simulink model "Lookup_verif"  (Simulink 7.2)
settings: Solver=ode45  StartTime=0.0  StopTime=10.0  RelTol=1e-3
settings Model: Creator=Romain  LastModifiedBy=Romain
settings OptimizationCC: ExpressionDepthLimit=128
settings DebuggingCC: SolverPrmCheckMsg=none  FcnCallInpInsideContextMsg=Enable All  StateNameClashWarn=none  StrictBusMsg=ErrorLevel1
settings CodeAppCC: CustomSymbolStrType=$N$R$M_T
settings GRTTargetCC: TargetFunctionLibrary=C89/C90 (ANSI)

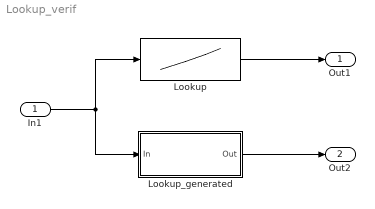
== system Lookup_verif ==
  In1 : Inport  OutDataTypeStr=double  DataType=double
  Lookup : Lookup  RequirementInfo={} %GIDa_7e2db0e9_94b6_4bd9_a9f6_4e499dfb9412  InputValues=[0 120 350 500]  Table=[1.0 1.0 0.3 0.3]
  Lookup_generated : Subsystem  TreatAsAtomicUnit=on
  Out1 : Outport
  Out2 : Outport  Port=2
  wires:
  In1/1 -> Lookup_generated/1(In), Lookup/1
  Lookup/1 -> Out1/1
  Lookup_generated/1(Out) -> Out2/1

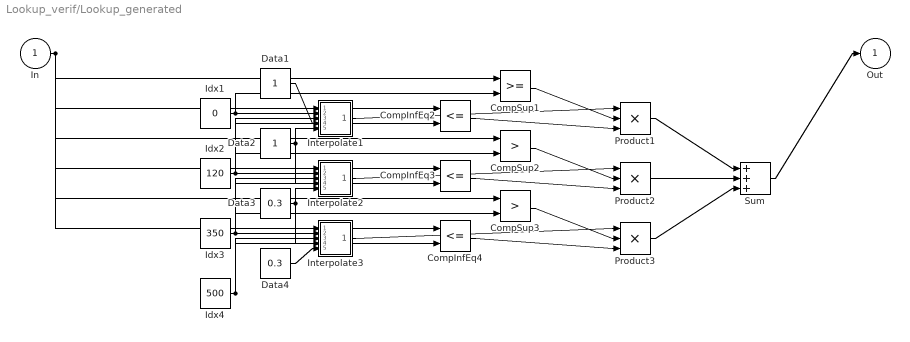
== system Lookup_verif/Lookup_generated ==
  In : Inport
  CompInfEq2 : RelationalOperator  Operator=<=  InputSameDT=on
  CompInfEq3 : RelationalOperator  Operator=<=  InputSameDT=on
  CompInfEq4 : RelationalOperator  Operator=<=  InputSameDT=on
  CompSup1 : RelationalOperator  InputSameDT=on
  CompSup2 : RelationalOperator  Operator=>  InputSameDT=on
  CompSup3 : RelationalOperator  Operator=>  InputSameDT=on
  Data1 : Constant
  Data2 : Constant
  Data3 : Constant  Value=0.3
  Data4 : Constant  Value=0.3
  Idx1 : Constant  Value=0
  Idx2 : Constant  Value=120
  Idx3 : Constant  Value=350
  Idx4 : Constant  Value=500
  Interpolate1 : Subsystem  TreatAsAtomicUnit=on
  Interpolate2 : Subsystem  TreatAsAtomicUnit=on
  Interpolate3 : Subsystem  TreatAsAtomicUnit=on
  Product1 : Product  Inputs=***  SaturateOnIntegerOverflow=on  RndMeth=Zero  OutDataTypeStr=Inherit: Same as first input
  Product2 : Product  Inputs=***  SaturateOnIntegerOverflow=on  RndMeth=Zero  OutDataTypeStr=Inherit: Same as first input
  Product3 : Product  Inputs=***  SaturateOnIntegerOverflow=on  RndMeth=Zero  OutDataTypeStr=Inherit: Same as first input
  Sum : Sum  Inputs=+++  SaturateOnIntegerOverflow=on  InputSameDT=on  OutDataTypeStr=Inherit: Same as first input
  Out : Outport
  wires:
  In/1 -> Interpolate1/1(InportIn), CompSup1/1, Interpolate2/1(InportIn), CompSup2/1, CompInfEq2/1, Interpolate3/1(InportIn), CompSup3/1, CompInfEq3/1, CompInfEq4/1
  Idx1/1 -> Interpolate1/2(InportIdx1), CompSup1/2
  Data1/1 -> Interpolate1/4(InportData1)
  Interpolate1/1(Out) -> Product1/1
  CompSup1/1 -> Product1/2
  CompInfEq2/1 -> Product1/3
  Product1/1 -> Sum/1
  Idx2/1 -> Interpolate2/2(InportIdx1), CompSup2/2, Interpolate1/3(InportIdx2), CompInfEq2/2
  Data2/1 -> Interpolate2/4(InportData1), Interpolate1/5(InportData2)
  Interpolate2/1(Out) -> Product2/1
  CompSup2/1 -> Product2/2
  CompInfEq3/1 -> Product2/3
  Product2/1 -> Sum/2
  Idx3/1 -> Interpolate3/2(InportIdx1), CompSup3/2, Interpolate2/3(InportIdx2), CompInfEq3/2
  Data3/1 -> Interpolate3/4(InportData1), Interpolate2/5(InportData2)
  Interpolate3/1(Out) -> Product3/1
  CompSup3/1 -> Product3/2
  CompInfEq4/1 -> Product3/3
  Product3/1 -> Sum/3
  Idx4/1 -> Interpolate3/3(InportIdx2), CompInfEq4/2
  Data4/1 -> Interpolate3/5(InportData2)
  Sum/1 -> Out/1

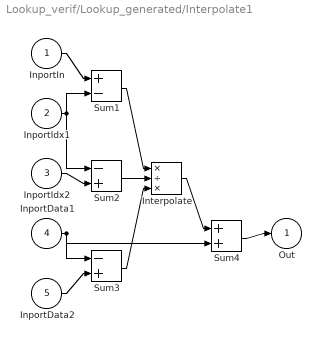
== system Lookup_verif/Lookup_generated/Interpolate1 ==
  InportIn : Inport
  InportIdx1 : Inport  Port=2
  InportIdx2 : Inport  Port=3
  InportData1 : Inport  Port=4
  InportData2 : Inport  Port=5
  Interpolate : Product  Inputs=*/*  SaturateOnIntegerOverflow=on  RndMeth=Zero  InputSameDT=on  OutDataTypeStr=Inherit: Same as first input
  Sum1 : Sum  Inputs=+-  SaturateOnIntegerOverflow=on  InputSameDT=on  OutDataTypeStr=Inherit: Same as first input
  Sum2 : Sum  Inputs=-+  SaturateOnIntegerOverflow=on  InputSameDT=on  OutDataTypeStr=Inherit: Same as first input
  Sum3 : Sum  Inputs=-+  SaturateOnIntegerOverflow=on  InputSameDT=on  OutDataTypeStr=Inherit: Same as first input
  Sum4 : Sum  SaturateOnIntegerOverflow=on  InputSameDT=on  OutDataTypeStr=Inherit: Same as first input
  Out : Outport
  wires:
  InportIn/1 -> Sum1/1
  InportIdx1/1 -> Sum1/2, Sum2/1
  InportIdx2/1 -> Sum2/2
  InportData1/1 -> Sum3/1, Sum4/2
  InportData2/1 -> Sum3/2
  Sum1/1 -> Interpolate/1
  Sum2/1 -> Interpolate/2
  Sum3/1 -> Interpolate/3
  Interpolate/1 -> Sum4/1
  Sum4/1 -> Out/1

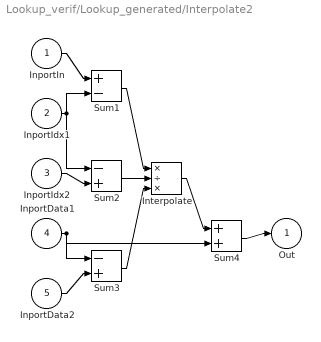
== system Lookup_verif/Lookup_generated/Interpolate2 ==
  InportIn : Inport
  InportIdx1 : Inport  Port=2
  InportIdx2 : Inport  Port=3
  InportData1 : Inport  Port=4
  InportData2 : Inport  Port=5
  Interpolate : Product  Inputs=*/*  SaturateOnIntegerOverflow=on  RndMeth=Zero  InputSameDT=on  OutDataTypeStr=Inherit: Same as first input
  Sum1 : Sum  Inputs=+-  SaturateOnIntegerOverflow=on  InputSameDT=on  OutDataTypeStr=Inherit: Same as first input
  Sum2 : Sum  Inputs=-+  SaturateOnIntegerOverflow=on  InputSameDT=on  OutDataTypeStr=Inherit: Same as first input
  Sum3 : Sum  Inputs=-+  SaturateOnIntegerOverflow=on  InputSameDT=on  OutDataTypeStr=Inherit: Same as first input
  Sum4 : Sum  SaturateOnIntegerOverflow=on  InputSameDT=on  OutDataTypeStr=Inherit: Same as first input
  Out : Outport
  wires:
  InportIn/1 -> Sum1/1
  InportIdx1/1 -> Sum1/2, Sum2/1
  InportIdx2/1 -> Sum2/2
  InportData1/1 -> Sum3/1, Sum4/2
  InportData2/1 -> Sum3/2
  Sum1/1 -> Interpolate/1
  Sum2/1 -> Interpolate/2
  Sum3/1 -> Interpolate/3
  Interpolate/1 -> Sum4/1
  Sum4/1 -> Out/1

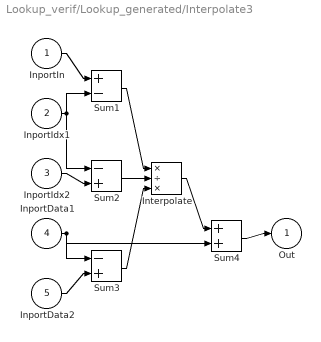
== system Lookup_verif/Lookup_generated/Interpolate3 ==
  InportIn : Inport
  InportIdx1 : Inport  Port=2
  InportIdx2 : Inport  Port=3
  InportData1 : Inport  Port=4
  InportData2 : Inport  Port=5
  Interpolate : Product  Inputs=*/*  SaturateOnIntegerOverflow=on  RndMeth=Zero  InputSameDT=on  OutDataTypeStr=Inherit: Same as first input
  Sum1 : Sum  Inputs=+-  SaturateOnIntegerOverflow=on  InputSameDT=on  OutDataTypeStr=Inherit: Same as first input
  Sum2 : Sum  Inputs=-+  SaturateOnIntegerOverflow=on  InputSameDT=on  OutDataTypeStr=Inherit: Same as first input
  Sum3 : Sum  Inputs=-+  SaturateOnIntegerOverflow=on  InputSameDT=on  OutDataTypeStr=Inherit: Same as first input
  Sum4 : Sum  SaturateOnIntegerOverflow=on  InputSameDT=on  OutDataTypeStr=Inherit: Same as first input
  Out : Outport
  wires:
  InportIn/1 -> Sum1/1
  InportIdx1/1 -> Sum1/2, Sum2/1
  InportIdx2/1 -> Sum2/2
  InportData1/1 -> Sum3/1, Sum4/2
  InportData2/1 -> Sum3/2
  Sum1/1 -> Interpolate/1
  Sum2/1 -> Interpolate/2
  Sum3/1 -> Interpolate/3
  Interpolate/1 -> Sum4/1
  Sum4/1 -> Out/1
